simulink model "pendulum_sim"  (R2016a)
settings: Solver=ode45  StartTime=0.0  StopTime=300  RelTol=1e-3
InitFcn:
  | param
undefined symbols (not defined in the file or in its folder): drawPendulum, P, pendulum_ctrl_alt1
settings Model: Creator=beard  LastModifiedBy=tmclain
settings DataIOCC: LimitDataPoints=on  SaveFormat=Array  SignalLoggingSaveFormat=ModelDataLogs
settings OptimizationCC: ExpressionDepthLimit=2147483647  InitFltsAndDblsToZero=on
settings DebuggingCC: UnderspecifiedInitializationDetection=Classic  MergeDetectMultiDrivingBlocksExec=none  SolverPrmCheckMsg=warning  FcnCallInpInsideContextMsg=UseLocalSettings  StateNameClashWarn=warning
settings HardwareCC: ProdBitPerPointer=32  ProdLargestAtomicFloat=None  ProdIntDivRoundTo=Undefined  ProdEndianess=Unspecified  ProdWordSize=32  ProdHWDeviceType=32-bit Generic
settings ModelReferenceCC: PropagateSignalLabelsOutOfModel=off
settings GRTTargetCC: CombineOutputUpdateFcns=off  GRTInterface=on
settings ConfigComp: CovModelRefEnable=Off

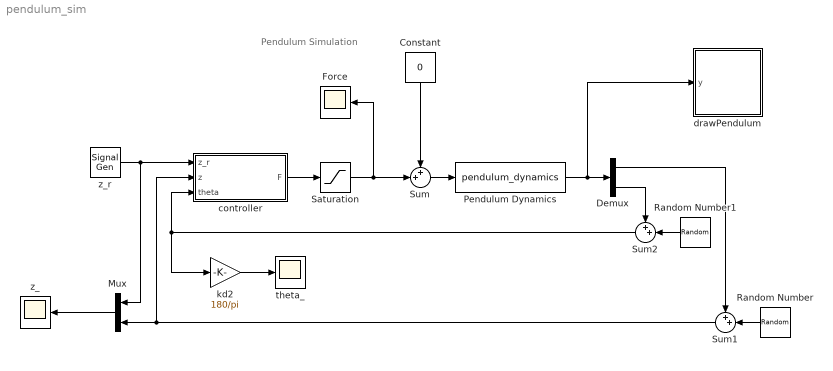
== system pendulum_sim ==
  note: Pendulum Simulation
  Constant : Constant  Value=0
  Demux : Demux  Outputs=2
  Force : Scope
  Mux : Mux  Inputs=2
  Pendulum Dynamics : S-Function  FunctionName=pendulum_dynamics  Parameters=P  SFunctionDeploymentMode=off  EnableBusSupport=off
  Random Number : RandomNumber  Variance=.001^2  SampleTime=P.Ts
  Random Number1 : RandomNumber  Variance=.001^2  SampleTime=P.Ts
  Saturation : Saturate  UpperLimit=10000  LowerLimit=-10000
  Sum : Sum  Inputs=++|
  Sum1 : Sum  Inputs=++|
  Sum2 : Sum  Inputs=++|
  controller : Subsystem
  drawPendulum : Subsystem
      mask Display: image(imread('tv.jpg'))
  kd2 : Gain  Gain=180/pi
  theta_ : Scope
  z_ : Scope
  z_r : SignalGenerator  WaveForm=square  Frequency=.025
  wires:
  Pendulum Dynamics/1 -> Demux/1, drawPendulum/1(y)
  controller/1(F) -> Saturation/1
  Saturation/1 -> Sum/2, Force/1
  z_r/1 -> Mux/1, controller/1(z_r)
  Mux/1 -> z_/1
  kd2/1 -> theta_/1
  Sum/1 -> Pendulum Dynamics/1
  Sum1/1 -> controller/2(z), Mux/2
  Demux/1 -> Sum1/1
  Sum2/1 -> kd2/1, controller/3(theta)
  Demux/2 -> Sum2/1
  Random Number/1 -> Sum1/2
  Random Number1/1 -> Sum2/2
  Constant/1 -> Sum/1

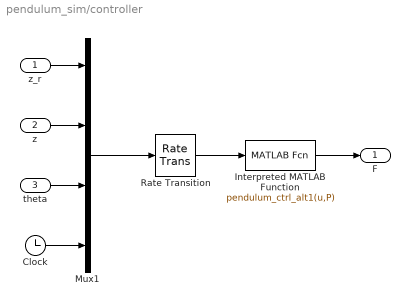
== system pendulum_sim/controller ==
  z_r : Inport
  z : Inport  Port=2
  theta : Inport  Port=3
  Clock : Clock
  Interpreted MATLAB Function : MATLABFcn  MATLABFcn=pendulum_ctrl_alt1(u,P)  OutputDimensions=1
  Mux1 : Mux
  Rate Transition : RateTransition  OutPortSampleTime=P.Ts
  F : Outport
  wires:
  Mux1/1 -> Rate Transition/1
  z_r/1 -> Mux1/1
  Clock/1 -> Mux1/4
  Rate Transition/1 -> Interpreted MATLAB Function/1
  theta/1 -> Mux1/3
  z/1 -> Mux1/2
  Interpreted MATLAB Function/1 -> F/1

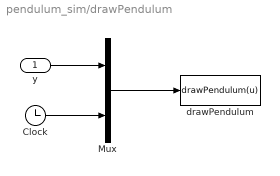
== system pendulum_sim/drawPendulum ==
  y : Inport
  Clock : Clock
  Mux : Mux  Inputs=2
  drawPendulum : MATLABFcn  MATLABFcn=drawPendulum(u)  OutputDimensions=0  SampleTime=0.1
  wires:
  Mux/1 -> drawPendulum/1
  y/1 -> Mux/1
  Clock/1 -> Mux/2
